simulink model "on_grid"  (R2015b)
settings: Solver=VariableStepAuto  StartTime=0.0  StopTime=2  RelTol=1e-3
InitFcn:
  | Ts_Power=0.5e-4;
  | Ts_Control=50e-4;
  | Ts=Ts_Power;
undefined symbols (not defined in the file): level
libraries: powerlib_extras x28, powerlib x24, powerlib_meascontrol x8, simulink x2
settings Model: Creator=fujitsu  LastModifiedBy=fujitsu

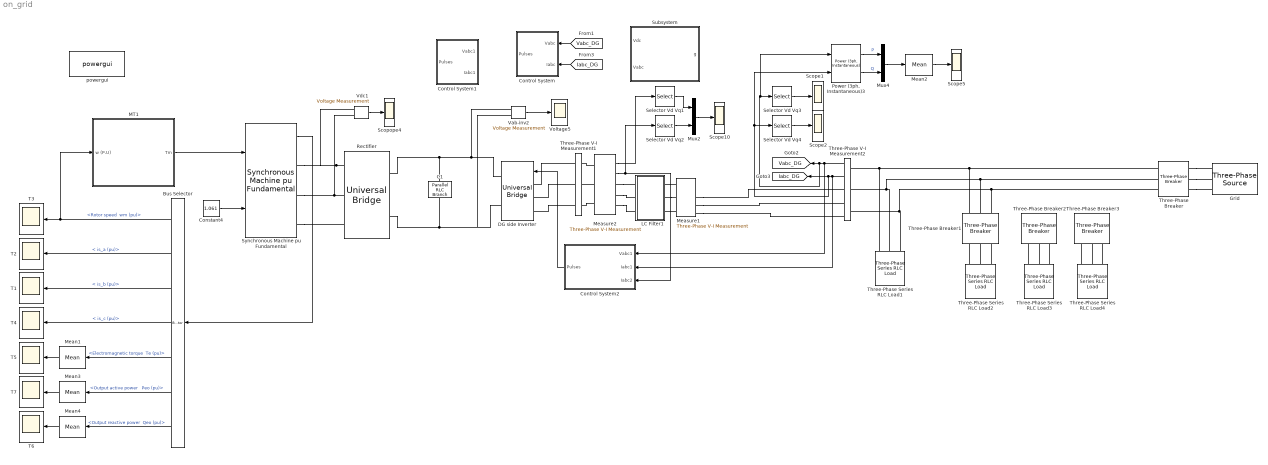
== system on_grid ==
  Bus Selector : BusSelector  OutputSignals="Mechanical.Rotor speed  wm (pu),Stator current. is_a (pu),Stator current. is_b (pu),Stator current. is_c (pu),Mechanical.Electromagnetic torque  Te (pu),Output active power   Peo (pu),Output reactive power  Qeo (pu)"
  C1 : powerlib/Elements/Parallel RLC Branch  LConnTagsString=a  RConnTagsString=__new0  BranchType=C  Resistance=inf  Inductance=inf  SetiL0=off  InitialCurrent=0  Capacitance=5000e-5  Setx0=off  InitialVoltage=0  Measurements=None
  Constant4 : Constant  Value=1.061
  Control System : Subsystem
  Control System1 : Subsystem
  Control System2 : Subsystem
      mask Display: fprintf('desired performance')
  DG side Inverter : powerlib/Power Electronics/Universal Bridge  Arms=3  SnubberResistance=10000  SnubberCapacitance=inf  Device=IGBT / Diodes  Ron=1e-4  Lon=0  ForwardVoltages="[  1  1  ]"  ForwardVoltage=.8  GTOparameters=[ 10e-6 , 20e-6 ]  IGBTparameters=[ 1e-6 , 2e-6 ]  Measurements=None  Measurements_2=None  converterType=Rectifier
  Grid : powerlib/Electrical Sources/Three-Phase Source  InternalConnection=Yg  VoltagePhases=off  Voltage=380  PhaseAngle=0  Voltage_phases=[25e3 25e3 25e3]/sqrt(3)  PhaseAngles_phases=[0 -120 +120]  Frequency=50  NonIdealSource=on  SpecifyImpedance=off  Resistance=0.02  Inductance=0.3e-3  ShortCircuitLevel=100e6  BaseVoltage=25e3  XRratio=7  BusType=swing  Pref=0  Qref=0  Prefabc=[10e3, 10e3, 10e3]  Qrefabc=[0, 0, 0]  Qmin=-inf  Qmax=inf
  LC Filter1 : Subsystem
  MT1 : Subsystem
  Mean{1..4} (4 alike) : powerlib_meascontrol/Measurements/Mean  Freq=50  Vinit=0  Ts=5e-6
  Measure1 : powerlib/Measurements/Three-Phase V-I Measurement  VoltageMeasurement=phase-to-phase  SetLabelV=off  LabelV=V1  Vpu=off  VpuLL=off  CurrentMeasurement=yes  SetLabelI=off  LabelI=I1  Ipu=off  Pbase=10e3  Vbase=400  OutputType=Magnitude  PhasorSimulation=off  PSBequivalent=0
  Measure2 : powerlib/Measurements/Three-Phase V-I Measurement  VoltageMeasurement=phase-to-phase  SetLabelV=off  LabelV=V1  Vpu=off  VpuLL=on  CurrentMeasurement=yes  SetLabelI=off  LabelI=I1  Ipu=on  Pbase=30e3  Vbase=380  OutputType=Magnitude  PhasorSimulation=off  PSBequivalent=0
  Mux2 : Mux  Inputs=2
  Mux4 : Mux  Inputs=2
  "Power (3ph, Instantaneous)3" : powerlib_meascontrol/Measurements/Power (3ph, Instantaneous)
  Rectifier : powerlib/Power Electronics/Universal Bridge  Arms=3  SnubberResistance=50  SnubberCapacitance=0.1e-6  Device=Diodes  Ron=1e-3  Lon=0  ForwardVoltages="[  0.8  0.8  ]"  ForwardVoltage=.7  GTOparameters=[ 10e-6 , 20e-6 ]  IGBTparameters=[ 1e-6 , 2e-6 ]  Measurements=Device currents  Measurements_2=None  converterType=Rectifier
  Scope{1..2,5,10} (4 alike) : Scope
  Scopope4 : Scope
  Selector Vd Vq{1..4} (4 alike) : Selector  InputPortWidth=3  IndexOptions=Index vector (dialog)  Indices=[1]  OutputSizes=1
  Subsystem : Subsystem  mask{kp=0.0001, ki=5}
      mask Display: fprintf('both on-grid & off-grid')
  Synchronous Machine pu Fundamental : powerlib/Machines/Synchronous Machine pu Fundamental  PresetModel=No  MechanicalLoad=Mechanical power Pm  ShowDetailedParameters=on  RotorType=Salient-pole  Units=per unit fundamental parameters  MeasurementBus=off  NominalParameters="[ 60e3  550 1600]"  Stator="[ 0.2503  0.114  0.6875  0.6875 ]"  Field="[ 1  10e15/(100*pi)]"  Dampers2=[0.0652, 0.5134, 0.0287, 0.2553, 7.765e-3, 0.9167 ]  Dampers1="[ 1.17E-02  0.182  1.97E-02  0.384 ]"  Mechanical=[ 6 0 2]  PolePairs=20  InitialConditions="[ 0  0  0  0  0  0  0  0  1 ]"  SetSaturation=off  Saturation=[0.6404,0.7127,0.8441,0.9214,0.9956,1.082,1.19,1.316,1.457;0.7,0.7698,0.8872,0.9466,0.9969,1.046,1.1,1.151,1.201]  LoadFlowParameters=[1,0,0,0,0]  TsPowergui=0  TsBlock=-1  IterativeModel=Trapezoidal non iterative  BusType=swing  Pref=0  Qref=0  Qmin=-inf  Qmax=inf  PLF=0  QLF=0
  T{1..7} (7 alike) : Scope
  Three-Phase Series RLC Load1 : powerlib/Elements/Three-Phase Series RLC Load  LConnTagsString=A|B|C  Configuration=Y (grounded)  NominalVoltage=380  Vabc=[1e3 1e3 1e3]  Vabcp=[1e3 1e3 1e3]  NominalFrequency=50  UnbalancedPower=off  ActivePower=1e3  InductivePower=0  CapacitivePower=0  Pabc=[10e3 9e3 11e3]  QLabc=[100 90 110]  QCabc=[100 90 110]  Pabcp=[10e3 9e3 11e3]  QLabcp=[100 90 110]  QCabcp=[100 90 110]  Measurements=None  LoadType=constant Z
  Three-Phase Series RLC Load2 : powerlib/Elements/Three-Phase Series RLC Load  LConnTagsString=A|B|C  Configuration=Y (grounded)  NominalVoltage=380  Vabc=[1e3 1e3 1e3]  Vabcp=[1e3 1e3 1e3]  NominalFrequency=50  UnbalancedPower=off  ActivePower=50e3  InductivePower=0  CapacitivePower=0  Pabc=[10e3 9e3 11e3]  QLabc=[100 90 110]  QCabc=[100 90 110]  Pabcp=[10e3 9e3 11e3]  QLabcp=[100 90 110]  QCabcp=[100 90 110]  Measurements=None  LoadType=constant Z
  Three-Phase Series RLC Load3 : powerlib/Elements/Three-Phase Series RLC Load  LConnTagsString=A|B|C  Configuration=Y (grounded)  NominalVoltage=380  Vabc=[1e3 1e3 1e3]  Vabcp=[1e3 1e3 1e3]  NominalFrequency=50  UnbalancedPower=off  ActivePower=15e3  InductivePower=0  CapacitivePower=0  Pabc=[10e3 9e3 11e3]  QLabc=[100 90 110]  QCabc=[100 90 110]  Pabcp=[10e3 9e3 11e3]  QLabcp=[100 90 110]  QCabcp=[100 90 110]  Measurements=None  LoadType=constant Z
  Three-Phase Series RLC Load4 : powerlib/Elements/Three-Phase Series RLC Load  LConnTagsString=A|B|C  Configuration=Y (grounded)  NominalVoltage=380  Vabc=[1e3 1e3 1e3]  Vabcp=[1e3 1e3 1e3]  NominalFrequency=50  UnbalancedPower=off  ActivePower=30e3  InductivePower=0  CapacitivePower=0  Pabc=[10e3 9e3 11e3]  QLabc=[100 90 110]  QCabc=[100 90 110]  Pabcp=[10e3 9e3 11e3]  QLabcp=[100 90 110]  QCabcp=[100 90 110]  Measurements=None  LoadType=constant Z
  Three-Phase V-I Measurement1 : powerlib/Measurements/Three-Phase V-I Measurement  VoltageMeasurement=no  SetLabelV=off  LabelV=Vabc  Vpu=on  VpuLL=off  CurrentMeasurement=no  SetLabelI=off  LabelI=Iabc  Ipu=on  Pbase=300e3  Vbase=208  OutputType=Complex  PhasorSimulation=off  PSBequivalent=0
  Three-Phase V-I Measurement2 : powerlib/Measurements/Three-Phase V-I Measurement  VoltageMeasurement=phase-to-phase  SetLabelV=off  LabelV=Vabc  Vpu=off  VpuLL=on  CurrentMeasurement=yes  SetLabelI=off  LabelI=Iabc  Ipu=on  Pbase=30e3  Vbase=380  OutputType=Complex  PhasorSimulation=off  PSBequivalent=0
  Three-Phase Breaker : powerlib/Elements/Three-Phase Breaker  InitialState=closed  SwitchA=on  SwitchB=on  SwitchC=on  SwitchTimes=[15]  External=off  BreakerResistance=0.01  SnubberResistance=1e6  SnubberCapacitance=inf  Measurements=None
  Three-Phase Breaker1 : powerlib/Elements/Three-Phase Breaker  InitialState=open  SwitchA=on  SwitchB=on  SwitchC=on  SwitchTimes=[1]  External=off  BreakerResistance=0.01  SnubberResistance=1e6  SnubberCapacitance=inf  Measurements=None
  Three-Phase Breaker2 : powerlib/Elements/Three-Phase Breaker  InitialState=closed  SwitchA=on  SwitchB=on  SwitchC=on  SwitchTimes=[6]  External=off  BreakerResistance=0.01  SnubberResistance=1e6  SnubberCapacitance=inf  Measurements=None
  Three-Phase Breaker3 : powerlib/Elements/Three-Phase Breaker  InitialState=open  SwitchA=on  SwitchB=on  SwitchC=on  SwitchTimes=[10 12]  External=off  BreakerResistance=0.01  SnubberResistance=1e6  SnubberCapacitance=inf  Measurements=None
  Vab-inv2 : powerlib/Measurements/Voltage Measurement  Tag=PoWeRsYsTeMmEaSuReMeNt  PhasorSimulation=off  OutputType=Magnitude  PSBequivalent=0
  Vdc1 : powerlib/Measurements/Voltage Measurement  Tag=PoWeRsYsTeMmEaSuReMeNt  PhasorSimulation=off  OutputType=Magnitude  PSBequivalent=0
  Voltage5 : Scope
  powergui : powerlib/powergui  SimulationMode=Discrete  SolverType=Tustin  SampleTime=5e-6  frequency=60  SPID=off  DisableSnubberDevices=off  DisableRonSwitches=off  DisableVfSwitches=off  SwTol=0  DisplayEquations=off  Interpol=off  ExternalGateDelay=off  methode=off  Ts=0  FunctionMessages=off  echomessages=off  HookPort=off  EnableUseOfTLC=off  x0status=blocks  frequencyindice=0  Pbase=100e6  ErrMax=0.0001  Iterations=50  UnitsV=kV  UnitsW=MW  buscounter=0  RestoreLinks=warning  ResistiveCurrentMeasurement=off  Frange=[0:2:500]  Ylog=off  Xlog=on  ShowGrid=off  save=off  variable=ZData  structure=Vs  ZoomFFT=on  StartTime=1/60  cycles=1  DisplayStyle=1  fundamental=60  FreqAxis=on  MaxFrequency=10000  frequencyindicesteady=1  RmsSteady=1  display=off
  tag scope: Iabc_DG=global, Vabc_DG=global
  wires:
  [Vabc_DG] -> Control System/1(Vabc)
  [Iabc_DG] -> Control System/2(Iabc)
  Three-Phase V-I Measurement2/1 -> Control System2/1(Vabc1), "Power (3ph, Instantaneous)3"/1, Selector Vd Vq3/1, [Vabc_DG]
  Three-Phase V-I Measurement2/2 -> Control System2/2(Iabc1), "Power (3ph, Instantaneous)3"/2, Selector Vd Vq4/1, [Iabc_DG]
  Vab-inv2/1 -> Voltage5/1
  Mux2/1 -> Scope10/1
  Selector Vd Vq1/1 -> Mux2/1
  Selector Vd Vq2/1 -> Mux2/2
  Measure2/1 -> Selector Vd Vq1/1
  Measure2/2 -> Control System2/3(Iabc2), Selector Vd Vq2/1
  Selector Vd Vq3/1 -> Scope1/1
  Selector Vd Vq4/1 -> Scope2/1
  Mux4/1 -> Mean2/1
  "Power (3ph, Instantaneous)3"/1 -> Mux4/1  "P"
  "Power (3ph, Instantaneous)3"/2 -> Mux4/2  "Q"
  Mean2/1 -> Scope5/1
  Control System2/1(Pulses) -> DG side Inverter/1
  MT1/1(Tm) -> Synchronous Machine pu Fundamental/1
  Synchronous Machine pu Fundamental/1 -> Bus Selector/1
  Constant4/1 -> Synchronous Machine pu Fundamental/2
  Vdc1/1 -> Scopope4/1
  Mean4/1 -> T6/1
  Bus Selector/1 -> MT1/1(w (P.U)), T3/1  "<Rotor speed  wm (pu)>"
  Bus Selector/2 -> T2/1  "< is_a (pu)>"
  Bus Selector/3 -> T1/1  "< is_b (pu)>"
  Bus Selector/4 -> T4/1  "< is_c (pu)>"
  Bus Selector/5 -> Mean1/1  "<Electromagnetic torque  Te (pu)>"
  Mean1/1 -> T5/1
  Bus Selector/7 -> Mean4/1  "<Output reactive power  Qeo (pu)>"
  Bus Selector/6 -> Mean3/1  "<Output active power   Peo (pu)>"
  Mean3/1 -> T7/1
  connections:
  Vab-inv2/LConn2 -- DG side Inverter/RConn2 -- Rectifier/RConn2 -- C1/RConn1
  Measure1/RConn2 -- Three-Phase V-I Measurement2/RConn2
  Measure1/RConn3 -- Three-Phase V-I Measurement2/RConn3
  Measure1/RConn1 -- Three-Phase V-I Measurement2/RConn1
  Three-Phase V-I Measurement1/RConn1 -- DG side Inverter/LConn1
  Three-Phase V-I Measurement1/RConn2 -- DG side Inverter/LConn2
  Three-Phase V-I Measurement1/RConn3 -- DG side Inverter/LConn3
  Vab-inv2/LConn1 -- C1/LConn1 -- Rectifier/RConn1 -- DG side Inverter/RConn1
  Measure1/LConn1 -- LC Filter1/RConn1
  Measure1/LConn3 -- LC Filter1/RConn3
  Measure2/LConn2 -- Three-Phase V-I Measurement1/LConn2
  Measure2/LConn1 -- Three-Phase V-I Measurement1/LConn1
  Measure2/LConn3 -- Three-Phase V-I Measurement1/LConn3
  Measure2/RConn1 -- LC Filter1/LConn1
  Measure2/RConn2 -- LC Filter1/LConn2
  Measure2/RConn3 -- LC Filter1/LConn3
  LC Filter1/RConn2 -- Measure1/LConn2
  Three-Phase Breaker/RConn1 -- Grid/RConn1
  Three-Phase Breaker/RConn2 -- Grid/RConn2
  Three-Phase Breaker/RConn3 -- Grid/RConn3
  Three-Phase Breaker/LConn1 -- Three-Phase Breaker1/LConn3 -- Three-Phase Series RLC Load1/LConn1 -- Three-Phase V-I Measurement2/LConn1
  Three-Phase Breaker/LConn2 -- Three-Phase Breaker1/LConn2 -- Three-Phase V-I Measurement2/LConn2 -- Three-Phase Series RLC Load1/LConn2
  Three-Phase Breaker/LConn3 -- Three-Phase Breaker1/LConn1 -- Three-Phase V-I Measurement2/LConn3 -- Three-Phase Series RLC Load1/LConn3
  Three-Phase Series RLC Load2/LConn1 -- Three-Phase Breaker1/RConn3
  Three-Phase Series RLC Load2/LConn2 -- Three-Phase Breaker1/RConn2
  Three-Phase Series RLC Load2/LConn3 -- Three-Phase Breaker1/RConn1
  Three-Phase Series RLC Load3/LConn1 -- Three-Phase Breaker2/RConn3
  Three-Phase Series RLC Load3/LConn2 -- Three-Phase Breaker2/RConn2
  Three-Phase Series RLC Load3/LConn3 -- Three-Phase Breaker2/RConn1
  Three-Phase Series RLC Load4/LConn1 -- Three-Phase Breaker3/RConn3
  Three-Phase Series RLC Load4/LConn2 -- Three-Phase Breaker3/RConn2
  Three-Phase Series RLC Load4/LConn3 -- Three-Phase Breaker3/RConn1
  Rectifier/LConn1 -- Synchronous Machine pu Fundamental/RConn1 -- Vdc1/LConn1
  Vdc1/LConn2 -- Synchronous Machine pu Fundamental/RConn2 -- Rectifier/LConn2
  Synchronous Machine pu Fundamental/RConn3 -- Rectifier/LConn3

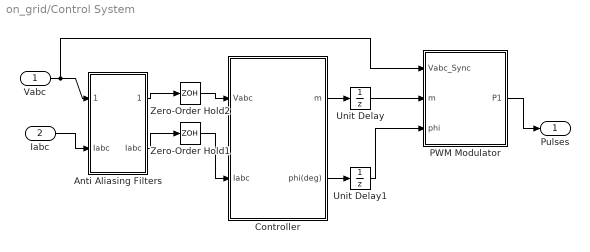
== system on_grid/Control System ==
  Vabc : Inport  PortDimensions=3
  Iabc : Inport  Port=2  PortDimensions=3
  Anti Aliasing Filters : Subsystem  mask(Anti-aliasing (2nd order lowpass)){Fc=2000, Ts=Ts_Power}
      mask prompts: Fc "Cut-off frequency (Hz):"; Ts "Sample time:"
  Controller : Subsystem
  PWM Modulator : Subsystem
  Unit Delay : UnitDelay  SampleTime=Ts_Control
  Unit Delay1 : UnitDelay  SampleTime=Ts_Control
  Zero-Order Hold1 : ZeroOrderHold  SampleTime=Ts_Control
  Zero-Order Hold2 : ZeroOrderHold  SampleTime=Ts_Control
  Pulses : Outport
  wires:
  Iabc/1 -> Anti Aliasing Filters/2("Iabc ")
  Anti Aliasing Filters/2(Iabc) -> Zero-Order Hold1/1
  Anti Aliasing Filters/1(" Vabc") -> Zero-Order Hold2/1
  Controller/1(m) -> Unit Delay/1
  Controller/2(phi(deg)) -> Unit Delay1/1
  Zero-Order Hold1/1 -> Controller/2(Iabc)
  Zero-Order Hold2/1 -> Controller/1(Vabc)
  Unit Delay1/1 -> PWM Modulator/3(phi)
  Unit Delay/1 -> PWM Modulator/2(m)
  Vabc/1 -> Anti Aliasing Filters/1(Vabc), PWM Modulator/1(Vabc_Sync)
  PWM Modulator/1(P1) -> Pulses/1

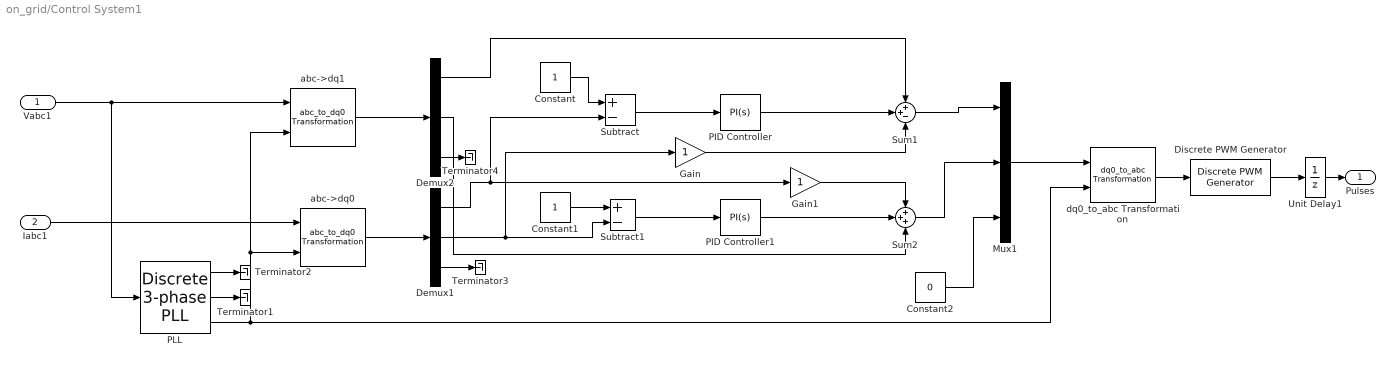
== system on_grid/Control System1 ==
  Vabc1 : Inport  PortDimensions=3
  Iabc1 : Inport  Port=2  PortDimensions=3
  " PLL" : powerlib_extras/Discrete  Control Blocks/Discrete 3-phase PLL  Fmin=45  Par_Init="[0  50]"  ParK=[60 1400]  Ts=Ts_Control  AGC=off
  Constant : Constant
  Constant1 : Constant
  Constant2 : Constant  Value=0
  Demux1 : Demux  Outputs=3
  Demux2 : Demux  Outputs=3
  Discrete PWM Generator : powerlib_extras/Discrete  Control Blocks/Discrete PWM Generator  GeneratorMode="3-arm  bridge (6 pulses)"  Fc=2000  Ts=5e-6  Internal=off  mIndex=0.4  Freq=60  Phase=0
  Gain : Gain
  Gain1 : Gain
  Mux1 : Mux  Inputs=3
  PID Controller : simulink/Continuous/PID Controller  Controller=PI  TimeDomain=Continuous-time  SampleTime=-1  IntegratorMethod=Forward Euler  FilterMethod=Forward Euler  Form=Parallel  UseFilter=on  ControllerParametersSource=internal  P=5  I=1  D=0  N=100  InitialConditionSource=internal  InitialConditionForIntegrator=0  InitialConditionForFilter=0  ExternalReset=none  LimitOutput=off  UpperSaturationLimit=inf  LowerSaturationLimit=-inf  LinearizeAsGain=on  AntiWindupMode=none  Kb=1  TrackingMode=off  Kt=1  PParamMin=[]  PParamMax=[]  IParamMin=[]  IParamMax=[]  DParamMin=[]  DParamMax=[]  NParamMin=[]  NParamMax=[]  KbParamMin=[]  KbParamMax=[]  KtParamMin=[]  KtParamMax=[]  POutMin=[]  POutMax=[]  IOutMin=[]  IOutMax=[]  DOutMin=[]  DOutMax=[]  NOutMin=[]  NOutMax=[]  KbOutMin=[]  KbOutMax=[]  KtOutMin=[]  KtOutMax=[]  IntegratorOutMin=[]  IntegratorOutMax=[]  FilterOutMin=[]  FilterOutMax=[]  SumOutMin=[]  SumOutMax=[]  SumI1OutMin=[]  SumI1OutMax=[]  SumI2OutMin=[]  SumI2OutMax=[]  SumI3OutMin=[]  SumI3OutMax=[]  SumDOutMin=[]  SumDOutMax=[]  SaturationOutMin=[]  SaturationOutMax=[]  IntegratorContinuousStateAttributes=''  IntegratorStateMustResolveToSignalObject=off  IntegratorRTWStateStorageClass=Auto  FilterContinuousStateAttributes=''  FilterStateMustResolveToSignalObject=off  FilterRTWStateStorageClass=Auto  DifferentiatorICPrevScaledInput=0  DifferentiatorOutMin=[]  DifferentiatorOutMax=[]
  PID Controller1 : simulink/Continuous/PID Controller  Controller=PI  TimeDomain=Continuous-time  SampleTime=-1  IntegratorMethod=Forward Euler  FilterMethod=Forward Euler  Form=Parallel  UseFilter=on  ControllerParametersSource=internal  P=1  I=5  D=0  N=100  InitialConditionSource=internal  InitialConditionForIntegrator=0  InitialConditionForFilter=0  ExternalReset=none  LimitOutput=off  UpperSaturationLimit=inf  LowerSaturationLimit=-inf  LinearizeAsGain=on  AntiWindupMode=none  Kb=1  TrackingMode=off  Kt=1  PParamMin=[]  PParamMax=[]  IParamMin=[]  IParamMax=[]  DParamMin=[]  DParamMax=[]  NParamMin=[]  NParamMax=[]  KbParamMin=[]  KbParamMax=[]  KtParamMin=[]  KtParamMax=[]  POutMin=[]  POutMax=[]  IOutMin=[]  IOutMax=[]  DOutMin=[]  DOutMax=[]  NOutMin=[]  NOutMax=[]  KbOutMin=[]  KbOutMax=[]  KtOutMin=[]  KtOutMax=[]  IntegratorOutMin=[]  IntegratorOutMax=[]  FilterOutMin=[]  FilterOutMax=[]  SumOutMin=[]  SumOutMax=[]  SumI1OutMin=[]  SumI1OutMax=[]  SumI2OutMin=[]  SumI2OutMax=[]  SumI3OutMin=[]  SumI3OutMax=[]  SumDOutMin=[]  SumDOutMax=[]  SaturationOutMin=[]  SaturationOutMax=[]  IntegratorContinuousStateAttributes=''  IntegratorStateMustResolveToSignalObject=off  IntegratorRTWStateStorageClass=Auto  FilterContinuousStateAttributes=''  FilterStateMustResolveToSignalObject=off  FilterRTWStateStorageClass=Auto  DifferentiatorICPrevScaledInput=0  DifferentiatorOutMin=[]  DifferentiatorOutMax=[]
  Subtract : Sum  Inputs=+-
  Subtract1 : Sum  Inputs=+-
  Sum1 : Sum  Inputs=++-
  Sum2 : Sum  Inputs=+++
  Terminator{1..4} (4 alike) : Terminator
  Unit Delay1 : UnitDelay  SampleTime=2e-6
  abc->dq0 : powerlib_extras/Measurements/abc_to_dq0 Transformation
  abc->dq1 : powerlib_extras/Measurements/abc_to_dq0 Transformation
  dq0_to_abc Transformation : powerlib_extras/Measurements/dq0_to_abc Transformation
  Pulses : Outport
  wires:
  Iabc1/1 -> abc->dq0/1
  " PLL"/1 -> Terminator2/1
  " PLL"/2 -> Terminator1/1
  Vabc1/1 -> " PLL"/1, abc->dq1/1
  " PLL"/3 -> dq0_to_abc Transformation/2, abc->dq1/2, abc->dq0/2
  abc->dq1/1 -> Demux2/1
  abc->dq0/1 -> Demux1/1
  Demux1/3 -> Terminator3/1
  Demux2/3 -> Terminator4/1
  Constant/1 -> Subtract/1
  Constant1/1 -> Subtract1/1
  Demux1/2 -> Gain/1, Subtract1/2
  Subtract1/1 -> PID Controller1/1
  Subtract/1 -> PID Controller/1
  PID Controller/1 -> Sum1/2
  Demux2/1 -> Sum1/1
  Gain/1 -> Sum1/3
  PID Controller1/1 -> Sum2/2
  Demux1/1 -> Subtract/2, Gain1/1
  Gain1/1 -> Sum2/1
  Demux2/2 -> Sum2/3
  Constant2/1 -> Mux1/3
  Sum1/1 -> Mux1/1
  Sum2/1 -> Mux1/2
  Discrete PWM Generator/1 -> Unit Delay1/1
  dq0_to_abc Transformation/1 -> Discrete PWM Generator/1
  Mux1/1 -> dq0_to_abc Transformation/1
  Unit Delay1/1 -> Pulses/1

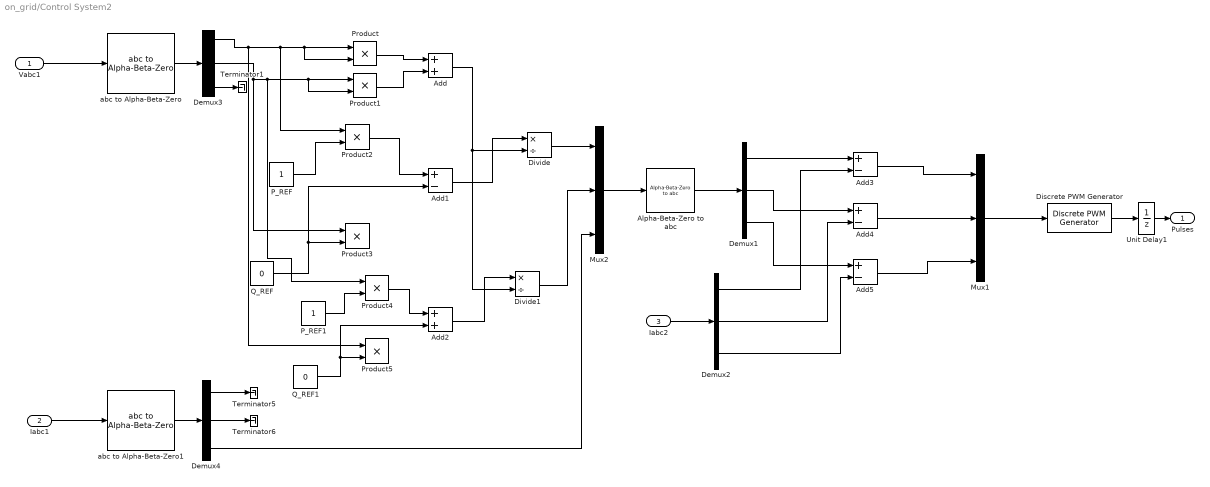
== system on_grid/Control System2 ==
  Vabc1 : Inport  PortDimensions=3
  Iabc1 : Inport  Port=2  PortDimensions=3
  Iabc2 : Inport  Port=3  PortDimensions=3
  Add : Sum
  Add{1,3..5} (4 alike) : Sum  Inputs=+-
  Add2 : Sum
  Alpha-Beta-Zero to abc : powerlib_meascontrol/Transformations/Alpha-Beta-Zero to abc
  Demux{1..4} (4 alike) : Demux  Outputs=3
  Discrete PWM Generator : powerlib_extras/Discrete  Control Blocks/Discrete PWM Generator  GeneratorMode="3-arm  bridge (6 pulses)"  Fc=8000  Ts=5e-6  Internal=off  mIndex=0.4  Freq=60  Phase=0
  Divide : Product  Inputs=*/
  Divide1 : Product  Inputs=*/
  Mux1 : Mux  Inputs=3
  Mux2 : Mux  Inputs=3
  P_REF : Constant
  P_REF1 : Constant
  Product{,1..5} (6 alike) : Product
  Q_REF : Constant  Value=0
  Q_REF1 : Constant  Value=0
  Terminator1 : Terminator
  Terminator5 : Terminator
  Terminator6 : Terminator
  Unit Delay1 : UnitDelay  SampleTime=5e-6
  abc to Alpha-Beta-Zero : powerlib_meascontrol/Transformations/abc to Alpha-Beta-Zero
  abc to Alpha-Beta-Zero1 : powerlib_meascontrol/Transformations/abc to Alpha-Beta-Zero
  Pulses : Outport
  wires:
  Unit Delay1/1 -> Pulses/1
  Discrete PWM Generator/1 -> Unit Delay1/1
  Vabc1/1 -> abc to Alpha-Beta-Zero/1
  abc to Alpha-Beta-Zero/1 -> Demux3/1
  Demux3/1 -> Product/1, Product/2, Product2/1, Product5/1
  Demux3/2 -> Product4/1, Product1/2, Product1/1, Product3/1
  Product/1 -> Add/1
  Product1/1 -> Add/2
  P_REF/1 -> Product2/2
  Q_REF/1 -> Add1/2, Product3/2
  Product2/1 -> Add1/1
  Add1/1 -> Divide/1
  Add/1 -> Divide1/2, Divide/2
  Divide/1 -> Mux2/1
  P_REF1/1 -> Product4/2
  Q_REF1/1 -> Add2/2, Product5/2
  Product4/1 -> Add2/1
  Add2/1 -> Divide1/1
  Divide1/1 -> Mux2/2
  Iabc1/1 -> abc to Alpha-Beta-Zero1/1
  abc to Alpha-Beta-Zero1/1 -> Demux4/1
  Demux4/3 -> Mux2/3
  Demux4/1 -> Terminator5/1
  Demux4/2 -> Terminator6/1
  Mux2/1 -> Alpha-Beta-Zero to abc/1
  Alpha-Beta-Zero to abc/1 -> Demux1/1
  Demux1/1 -> Add3/1
  Iabc2/1 -> Demux2/1
  Demux2/1 -> Add3/2
  Demux1/2 -> Add4/1
  Demux2/2 -> Add4/2
  Demux1/3 -> Add5/1
  Demux2/3 -> Add5/2
  Add3/1 -> Mux1/1
  Add4/1 -> Mux1/2
  Add5/1 -> Mux1/3
  Mux1/1 -> Discrete PWM Generator/1
  Demux3/3 -> Terminator1/1

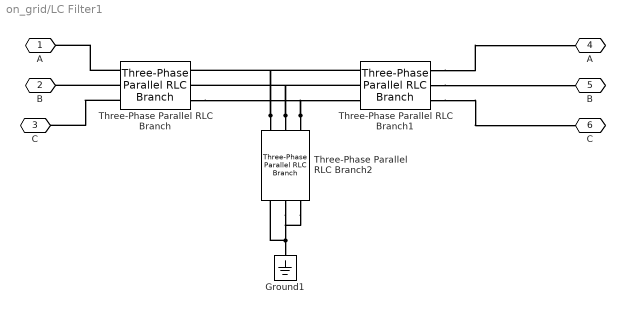
== system on_grid/LC Filter1 ==
  Ground1 : powerlib/Elements/Ground  LConnTagsString=a
  Three-Phase Parallel RLC Branch : powerlib/Elements/Three-Phase Parallel RLC Branch  LConnTagsString=A|B|C  RConnTagsString=A|B|C  BranchType=L  Resistance=1  Inductance=5.7e-3  Capacitance=1e-6  Measurements=None
  Three-Phase Parallel RLC Branch1 : powerlib/Elements/Three-Phase Parallel RLC Branch  LConnTagsString=A|B|C  RConnTagsString=A|B|C  BranchType=R  Resistance=0.00001  Inductance=5.7e-3  Capacitance=1e-6  Measurements=None
  Three-Phase Parallel RLC Branch2 : powerlib/Elements/Three-Phase Parallel RLC Branch  LConnTagsString=A|B|C  RConnTagsString=A|B|C  BranchType=C  Resistance=1  Inductance=5.7e-3  Capacitance=1000e-6  Measurements=None
  A : PMIOPort  Port=1  Side=Left
  B : PMIOPort  Port=2  Side=Left
  C : PMIOPort  Port=3  Side=Left
  "A " : PMIOPort  Port=4  Side=Right
  "B " : PMIOPort  Port=5  Side=Right
  "C " : PMIOPort  Port=6  Side=Right
  connections:
  Ground1/LConn1 -- Three-Phase Parallel RLC Branch2/RConn2 -- Three-Phase Parallel RLC Branch2/RConn1 -- Three-Phase Parallel RLC Branch2/RConn3
  Three-Phase Parallel RLC Branch1/RConn3 -- "C "/RConn1
  Three-Phase Parallel RLC Branch1/RConn2 -- "B "/RConn1
  Three-Phase Parallel RLC Branch1/RConn1 -- "A "/RConn1
  Three-Phase Parallel RLC Branch2/LConn3 -- Three-Phase Parallel RLC Branch1/LConn3 -- Three-Phase Parallel RLC Branch/RConn3
  Three-Phase Parallel RLC Branch2/LConn2 -- Three-Phase Parallel RLC Branch/RConn2 -- Three-Phase Parallel RLC Branch1/LConn2
  Three-Phase Parallel RLC Branch2/LConn1 -- Three-Phase Parallel RLC Branch/RConn1 -- Three-Phase Parallel RLC Branch1/LConn1
  Three-Phase Parallel RLC Branch/LConn3 -- C/RConn1
  Three-Phase Parallel RLC Branch/LConn2 -- B/RConn1
  Three-Phase Parallel RLC Branch/LConn1 -- A/RConn1

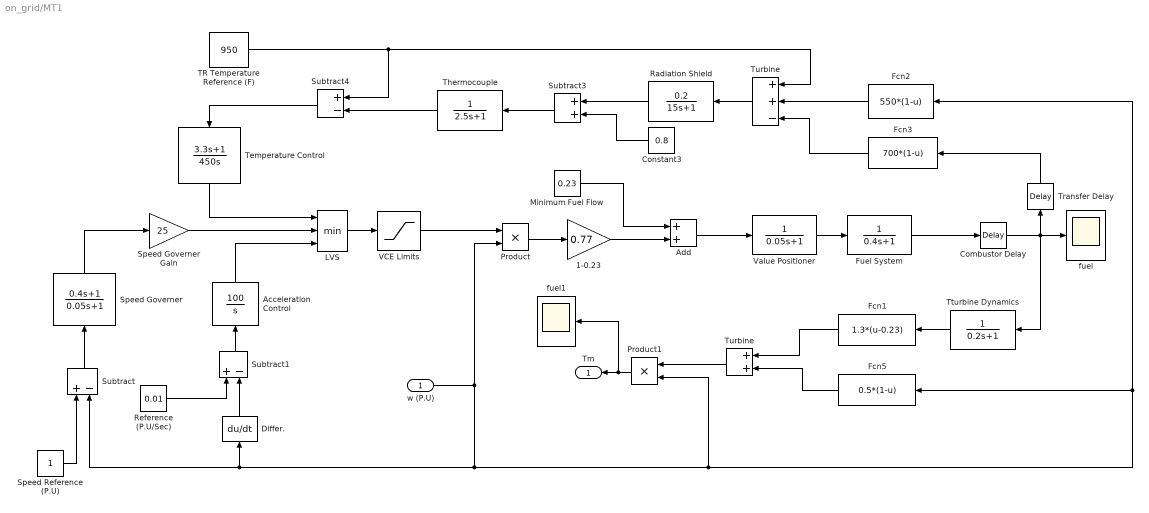
== system on_grid/MT1 ==
  w (P.U) : Inport
  1-0.23 : Gain  Gain=0.77
  Acceleration Control : TransferFcn  Numerator=[0 100]  Denominator=[1 0]
  Add : Sum
  Combustor Delay : TransportDelay  DelayTime=0.01
  Constant3 : Constant  Value=0.8
  Differ. : Derivative
  Fcn1 : Fcn  Expr=1.3*(u-0.23)
  Fcn2 : Fcn  Expr=550*(1-u)
  Fcn3 : Fcn  Expr=700*(1-u)
  Fcn5 : Fcn  Expr=0.5*(1-u)
  Fuel System : TransferFcn  Denominator=[0.4 1]
  LVS : MinMax  Inputs=3
  Minimum Fuel Flow : Constant  Value=0.23
  Product : Product  RndMeth=Zero
  Product1 : Product  RndMeth=Zero
  Radiation Shield : TransferFcn  Numerator=[0.2]  Denominator=[15 1]
  Reference (P.U/Sec) : Constant  Value=0.01
  Speed Governer : TransferFcn  Numerator=[0.4 1]  Denominator=[0.05 1]
  Speed Governer Gain : Gain  Gain=25
  Speed Reference (P.U) : Constant
  Subtract : Sum  Inputs=+-
  Subtract1 : Sum  Inputs=+-
  Subtract3 : Sum
  Subtract4 : Sum  Inputs=+-
  TR Temperature Reference (F) : Constant  Value=950
  Temperature Control : TransferFcn  Numerator=[3.3 1]  Denominator=[450 0]
  Thermocouple : TransferFcn  Denominator=[2.5 1]
  Transfer Delay : TransportDelay  DelayTime=0.04
  Tturbine Dynamics : TransferFcn  Denominator=[0.2 1]
  Turbine : Sum  Inputs=++-
  "Turbine " : Sum
  VCE Limits : Saturate  UpperLimit=1.5  LowerLimit=-0.1
  Value Positioner : TransferFcn  Denominator=[0.05 1]
  fuel : Scope
  fuel1 : Scope
  Tm : Outport
  wires:
  "Turbine "/1 -> Product1/1
  Product1/1 -> fuel1/1, Tm/1
  Fcn5/1 -> "Turbine "/2
  Fcn1/1 -> "Turbine "/1
  Tturbine Dynamics/1 -> Fcn1/1
  w (P.U)/1 -> Fcn2/1, Fcn5/1, Product1/2, Differ./1, Subtract/2, Product/2
  Speed Governer/1 -> Speed Governer Gain/1
  Temperature Control/1 -> LVS/1
  Subtract4/1 -> Temperature Control/1
  TR Temperature Reference (F)/1 -> Subtract4/1, Turbine/1
  Thermocouple/1 -> Subtract4/2
  Subtract3/1 -> Thermocouple/1
  Turbine/1 -> Radiation Shield/1
  Constant3/1 -> Subtract3/2
  Radiation Shield/1 -> Subtract3/1
  Fcn2/1 -> Turbine/2
  Fcn3/1 -> Turbine/3
  Transfer Delay/1 -> Fcn3/1
  LVS/1 -> VCE Limits/1
  Acceleration Control/1 -> LVS/3
  Subtract1/1 -> Acceleration Control/1
  Reference (P.U/Sec)/1 -> Subtract1/1
  Differ./1 -> Subtract1/2
  Speed Governer Gain/1 -> LVS/2
  Combustor Delay/1 -> Tturbine Dynamics/1, fuel/1, Transfer Delay/1
  Fuel System/1 -> Combustor Delay/1
  Value Positioner/1 -> Fuel System/1
  Add/1 -> Value Positioner/1
  Minimum Fuel Flow/1 -> Add/1
  1-0.23/1 -> Add/2
  Product/1 -> 1-0.23/1
  VCE Limits/1 -> Product/1
  Subtract/1 -> Speed Governer/1
  Speed Reference (P.U)/1 -> Subtract/1

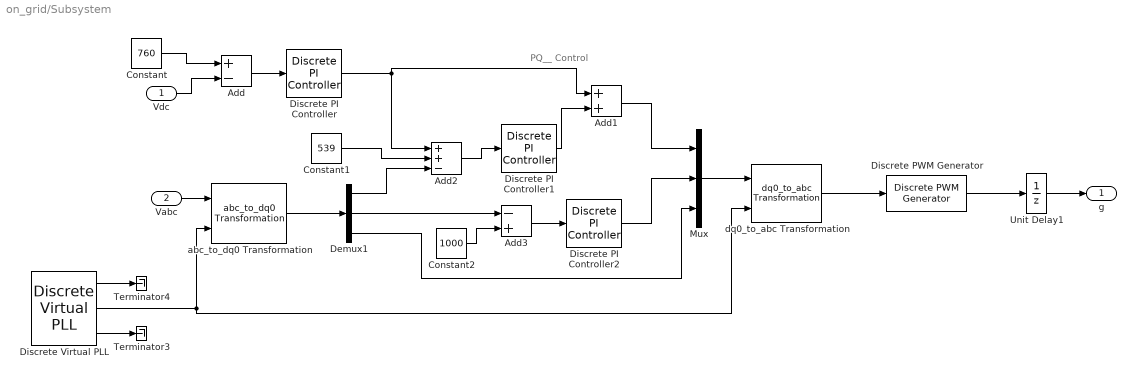
== system on_grid/Subsystem ==
  note: PQ__ Control
  Vdc : Inport
  Vabc : Inport  Port=2
  Add : Sum  Inputs=+-
  Add1 : Sum
  Add2 : Sum  Inputs=++-
  Add3 : Sum  Inputs=-+
  Constant : Constant  Value=760
  Constant1 : Constant  Value=539
  Constant2 : Constant  Value=1000
  Demux1 : Demux  Outputs=3
  Discrete PI Controller : powerlib_extras/Discrete  Control Blocks/Discrete PI Controller  Kp=kp  Ki=ki  Par_Limits=[1e6 -1e6]  Init=0  Ts=50e-6
  Discrete PI Controller1 : powerlib_extras/Discrete  Control Blocks/Discrete PI Controller  Kp=kp  Ki=ki  Par_Limits=[1e6 -1e6]  Init=0  Ts=50e-6
  Discrete PI Controller2 : powerlib_extras/Discrete  Control Blocks/Discrete PI Controller  Kp=kp  Ki=ki  Par_Limits=[1e6 -1e6]  Init=0  Ts=50e-6
  Discrete PWM Generator : powerlib_extras/Discrete  Control Blocks/Discrete PWM Generator  GeneratorMode="3-arm  bridge (6 pulses)"  Fc=2000  Ts=2e-6  Internal=off  mIndex=0.4  Freq=60  Phase=0
  Discrete Virtual PLL : powerlib_extras/Discrete  Control Blocks/Discrete Virtual PLL  Freq=50  Phase=0  Ts=50e-6
  Mux : Mux  Inputs=3
  Terminator3 : Terminator
  Terminator4 : Terminator
  Unit Delay1 : UnitDelay  SampleTime=2e-6
  abc_to_dq0 Transformation : powerlib_extras/Measurements/abc_to_dq0 Transformation
  dq0_to_abc Transformation : powerlib_extras/Measurements/dq0_to_abc Transformation
  g : Outport
  wires:
  Constant/1 -> Add/1
  Vdc/1 -> Add/2
  Add/1 -> Discrete PI Controller/1
  Discrete PI Controller/1 -> Add1/1, Add2/1
  Constant1/1 -> Add2/2
  Add2/1 -> Discrete PI Controller1/1
  Discrete PI Controller1/1 -> Add1/2
  Add1/1 -> Mux/1
  Vabc/1 -> abc_to_dq0 Transformation/1
  abc_to_dq0 Transformation/1 -> Demux1/1
  Demux1/1 -> Add2/3
  Demux1/2 -> Add3/1
  Constant2/1 -> Add3/2
  Add3/1 -> Discrete PI Controller2/1
  Discrete PI Controller2/1 -> Mux/2
  Demux1/3 -> Mux/3
  Discrete Virtual PLL/1 -> Terminator4/1
  Discrete Virtual PLL/3 -> Terminator3/1
  Discrete Virtual PLL/2 -> abc_to_dq0 Transformation/2, dq0_to_abc Transformation/2
  Mux/1 -> dq0_to_abc Transformation/1
  Discrete PWM Generator/1 -> Unit Delay1/1
  dq0_to_abc Transformation/1 -> Discrete PWM Generator/1
  Unit Delay1/1 -> g/1

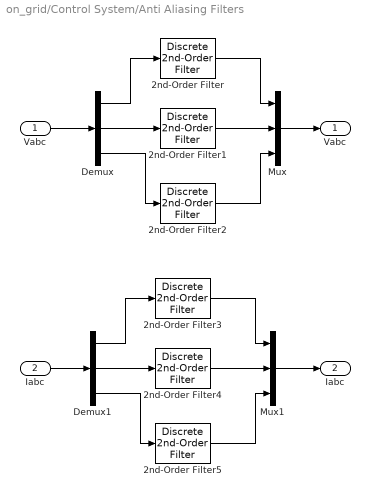
== system on_grid/Control System/Anti Aliasing Filters ==
  Vabc : Inport  PortDimensions=3
  "Iabc " : Inport  Port=2  PortDimensions=3
  2nd-Order Filter : powerlib_extras/Discrete  Control Blocks/Discrete  2nd-Order Filter  FilterType=Lowpass  Fo=Fc  Zeta=0.707  Ts=Ts  Initialize=off  Vac_Init=[0.8 -25 60]  Vdc_Init=-0.4  PlotResponse=off  param1=[1 120 0.1]
  2nd-Order Filter{1..5} (5 alike) : powerlib_extras/Discrete  Control Blocks/Discrete  2nd-Order Filter  FilterType=Lowpass  Fo=Fc  Zeta=0.707  Ts=Ts  Initialize=off  Vac_Init=[0.8 -25 60]  Vdc_Init=-0.4  PlotResponse=off  param1=[1 5000 0.1]
  Demux : Demux  Outputs=3
  Demux1 : Demux  Outputs=3
  Mux : Mux  Inputs=3
  Mux1 : Mux  Inputs=3
  " Vabc" : Outport
  Iabc : Outport  Port=2
  wires:
  "Iabc "/1 -> Demux1/1
  Demux1/2 -> 2nd-Order Filter4/1
  Demux1/3 -> 2nd-Order Filter5/1
  2nd-Order Filter5/1 -> Mux1/3
  2nd-Order Filter4/1 -> Mux1/2
  Mux1/1 -> Iabc/1
  2nd-Order Filter3/1 -> Mux1/1
  Demux1/1 -> 2nd-Order Filter3/1
  Demux/2 -> 2nd-Order Filter1/1
  Demux/3 -> 2nd-Order Filter2/1
  2nd-Order Filter2/1 -> Mux/3
  2nd-Order Filter1/1 -> Mux/2
  Mux/1 -> " Vabc"/1
  2nd-Order Filter/1 -> Mux/1
  Vabc/1 -> Demux/1
  Demux/1 -> 2nd-Order Filter/1

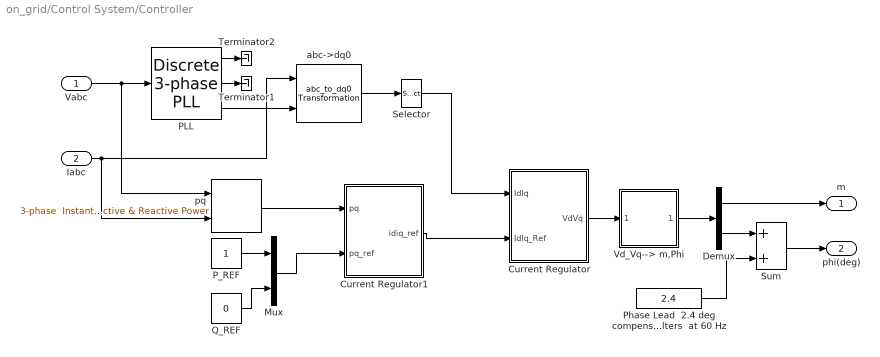
== system on_grid/Control System/Controller ==
  Vabc : Inport  PortDimensions=3
  Iabc : Inport  Port=2  PortDimensions=3
  " PLL" : powerlib_extras/Discrete  Control Blocks/Discrete 3-phase PLL  Fmin=750  Par_Init="[-500  1000]"  ParK=[60 1400]  Ts=Ts_Control  AGC=off
  Current Regulator : Subsystem  mask(Current Regulators){Kp=3, Ki=0.08, Kd=0, TcD=0.2e-3, Par_Limits=[1 -1], Init=[1 0], Ts=Ts_Control}
      mask prompts: Kp "Proportional gain (Kp):"; Ki "Integral gain (Ki):"; Kd "Derivative gain (Kd):"; TcD "Time constant for derivative (s):"; Par_Limits "Output limits: [ Upper   Lower ]"; Init "Output initial value:"; Ts "Sample time:"
      mask help:
      | Sign convention:
      | Id positive(+) flowing out of converter ==> Converter delivering real power = P positive(+)
      | Iq negative(-) flowing out of  converter (inductive current) ==> Converter delivering reactive power = Q positive(+)
  Current Regulator1 : Subsystem  mask(Current Regulators){Kp=5, Ki=0.07, Kd=0, TcD=0, Par_Limits=[1 -1], Init=[1 0], Ts=Ts_Control}
      mask prompts: Kp "Proportional gain (Kp):"; Ki "Integral gain (Ki):"; Kd "Derivative gain (Kd):"; TcD "Time constant for derivative (s):"; Par_Limits "Output limits: [ Upper   Lower ]"; Init "Output initial value:"; Ts "Sample time:"
      mask help:
      | Sign convention:
      | Id positive(+) flowing out of converter ==> Converter delivering real power = P positive(+)
      | Iq negative(-) flowing out of  converter (inductive current) ==> Converter delivering reactive power = Q positive(+)
  Demux : Demux  Outputs=2
  Mux : Mux  Inputs=2
  P_REF : Constant
  Phase Lead  2.4 deg compensating phase shift of anti-aliasing  filters  at 60 Hz : Constant  Value=2.4
  Q_REF : Constant  Value=0
  Selector : Selector  InputPortWidth=3  IndexOptions=Index vector (dialog)  Indices=[1 2]  OutputSizes=1
  Sum : Sum  SaturateOnIntegerOverflow=on  InputSameDT=on  OutDataTypeStr=Inherit: Same as first input
  Terminator1 : Terminator
  Terminator2 : Terminator
  Vd_Vq--> m,Phi : Subsystem
  abc->dq0 : powerlib_extras/Measurements/abc_to_dq0 Transformation
  pq : powerlib_extras/Measurements/3-phase  Instantaneous  Active & Reactive Power
  m : Outport
  phi(deg) : Outport  Port=2
  wires:
  " PLL"/1 -> Terminator2/1
  Sum/1 -> phi(deg)/1
  Phase Lead  2.4 deg compensating phase shift of anti-aliasing  filters  at 60 Hz/1 -> Sum/2
  Demux/2 -> Sum/1
  " PLL"/2 -> Terminator1/1
  abc->dq0/1 -> Selector/1
  Vd_Vq--> m,Phi/1(m_Phi) -> Demux/1
  Current Regulator/1(VdVq) -> Vd_Vq--> m,Phi/1(VdVq)
  Demux/1 -> m/1
  Vabc/1 -> " PLL"/1, pq/1
  " PLL"/3 -> abc->dq0/2
  Iabc/1 -> abc->dq0/1, pq/2
  Selector/1 -> Current Regulator/1(IdIq)
  Current Regulator1/1(idiq_ref) -> Current Regulator/2(IdIq_Ref)
  Mux/1 -> Current Regulator1/2(pq_ref)
  Q_REF/1 -> Mux/2
  P_REF/1 -> Mux/1
  pq/1 -> Current Regulator1/1(pq)

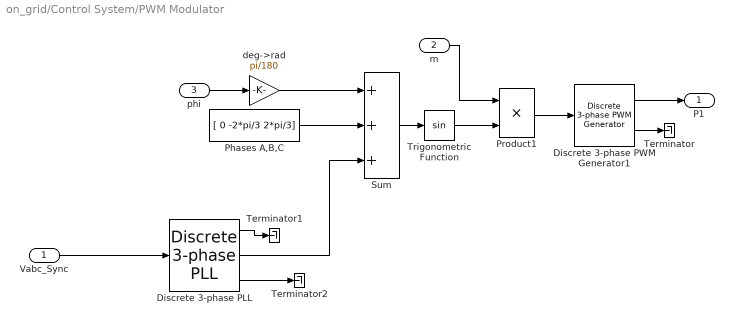
== system on_grid/Control System/PWM Modulator ==
  Vabc_Sync : Inport  PortDimensions=3
  m : Inport  Port=2  PortDimensions=1
  phi : Inport  Port=3  PortDimensions=1
  Discrete 3-phase PLL : powerlib_extras/Discrete  Control Blocks/Discrete 3-phase PLL  Fmin=55  Par_Init=[0 60]  ParK=[60 1400]  Ts=Ts_Power*2  AGC=off
  Discrete 3-phase PWM Generator1 : powerlib_extras/Discrete  Control Blocks/Discrete 3-phase PWM Generator  ModulatorType=2-level  ModulatorMode=Un-synchronized  nF=9  Fc=20e3  ModulatingSignals=off  m=0.8  Freq=1115  Phase=-14  Ts=Ts_Power
  Phases A,B,C : Constant  Value=[ 0 -2*pi/3 2*pi/3]
  Product1 : Product  SaturateOnIntegerOverflow=on  InputSameDT=on  OutDataTypeStr=Inherit: Same as first input
  Sum : Sum  Inputs=+++  SaturateOnIntegerOverflow=on  InputSameDT=on  OutDataTypeStr=Inherit: Same as first input
  Terminator : Terminator
  Terminator1 : Terminator
  Terminator2 : Terminator
  Trigonometric Function : Trigonometry
  deg->rad : Gain  Gain=pi/180  SaturateOnIntegerOverflow=on  OutDataTypeStr=Inherit: Same as input  ParamDataTypeStr=Inherit: Same as input
  P1 : Outport
  wires:
  Discrete 3-phase PLL/2 -> Sum/3
  Sum/1 -> Trigonometric Function/1
  Trigonometric Function/1 -> Product1/2
  m/1 -> Product1/1
  Product1/1 -> Discrete 3-phase PWM Generator1/1
  Discrete 3-phase PWM Generator1/1 -> P1/1
  Discrete 3-phase PWM Generator1/2 -> Terminator/1
  Discrete 3-phase PLL/3 -> Terminator2/1
  Vabc_Sync/1 -> Discrete 3-phase PLL/1
  deg->rad/1 -> Sum/1
  phi/1 -> deg->rad/1
  Phases A,B,C/1 -> Sum/2
  Discrete 3-phase PLL/1 -> Terminator1/1

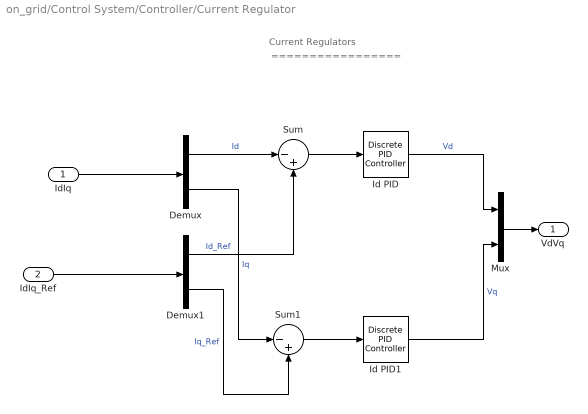
== system on_grid/Control System/Controller/Current Regulator ==
  note: =================
  note: Current Regulators
  IdIq : Inport  PortDimensions=2
  IdIq_Ref : Inport  Port=2  PortDimensions=2
  Demux : Demux  Outputs=2
  Demux1 : Demux  Outputs=2
  Id PID : powerlib_extras/Discrete  Control Blocks/Discrete PID Controller  Kp=Kp  Ki=Ki  Kd=Kd  TcD=TcD  Par_Limits=Par_Limits  Init=Init(1)  Ts=Ts
  Id PID1 : powerlib_extras/Discrete  Control Blocks/Discrete PID Controller  Kp=Kp  Ki=Ki  Kd=Kd  TcD=TcD  Par_Limits=Par_Limits  Init=Init(2)  Ts=Ts
  Mux : Mux  Inputs=2
  Sum : Sum  Inputs=|-+  SaturateOnIntegerOverflow=on  InputSameDT=on  OutDataTypeStr=Inherit: Same as first input
  Sum1 : Sum  Inputs=|-+  SaturateOnIntegerOverflow=on  InputSameDT=on  OutDataTypeStr=Inherit: Same as first input
  VdVq : Outport
  wires:
  IdIq_Ref/1 -> Demux1/1
  Mux/1 -> VdVq/1
  Sum/1 -> Id PID/1
  Demux1/2 -> Sum1/2  "Iq_Ref"
  Sum1/1 -> Id PID1/1
  Demux/2 -> Sum1/1  "Iq"
  Demux1/1 -> Sum/2  "Id_Ref"
  Demux/1 -> Sum/1  "Id"
  Id PID/1 -> Mux/1  "Vd"
  Id PID1/1 -> Mux/2  "Vq"
  IdIq/1 -> Demux/1

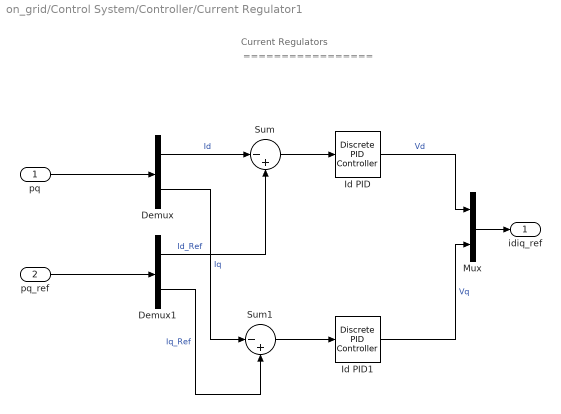
== system on_grid/Control System/Controller/Current Regulator1 ==
  note: =================
  note: Current Regulators
  pq : Inport  PortDimensions=2
  pq_ref : Inport  Port=2  PortDimensions=2
  Demux : Demux  Outputs=2
  Demux1 : Demux  Outputs=2
  Id PID : powerlib_extras/Discrete  Control Blocks/Discrete PID Controller  Kp=Kp  Ki=Ki  Kd=Kd  TcD=TcD  Par_Limits=Par_Limits  Init=Init(1)  Ts=Ts
  Id PID1 : powerlib_extras/Discrete  Control Blocks/Discrete PID Controller  Kp=Kp  Ki=Ki  Kd=Kd  TcD=TcD  Par_Limits=Par_Limits  Init=Init(2)  Ts=Ts
  Mux : Mux  Inputs=2
  Sum : Sum  Inputs=|-+  SaturateOnIntegerOverflow=on  InputSameDT=on  OutDataTypeStr=Inherit: Same as first input
  Sum1 : Sum  Inputs=|-+  SaturateOnIntegerOverflow=on  InputSameDT=on  OutDataTypeStr=Inherit: Same as first input
  idiq_ref : Outport
  wires:
  pq_ref/1 -> Demux1/1
  Mux/1 -> idiq_ref/1
  Sum/1 -> Id PID/1
  Demux1/2 -> Sum1/2  "Iq_Ref"
  Sum1/1 -> Id PID1/1
  Demux/2 -> Sum1/1  "Iq"
  Demux1/1 -> Sum/2  "Id_Ref"
  Demux/1 -> Sum/1  "Id"
  Id PID/1 -> Mux/1  "Vd"
  Id PID1/1 -> Mux/2  "Vq"
  pq/1 -> Demux/1

== system on_grid/Control System/Controller/Vd_Vq--> m,Phi ==
  VdVq : Inport
  Fcn3 : Fcn  Expr=sqrt(u[1]*u[1]+u[2]*u[2])
  Fcn4 : Fcn  Expr=atan2(u[2]+1e-6,u[1])*180/pi
  Mux2 : Mux  Inputs=2
  m_Phi : Outport
  wires:
  Fcn4/1 -> Mux2/2
  Mux2/1 -> m_Phi/1
  Fcn3/1 -> Mux2/1
  VdVq/1 -> Fcn4/1, Fcn3/1
